simulink model "GCU_Model_genCode"  (R2018a)
settings: Solver=FixedStepDiscrete  StartTime=0.0  StopTime=20  FixedStep=0.0001  RelTol=1e-3  EnableMultiTasking=on
undefined symbols (not defined in the file): ConversionGainVector, ConversionOffsetVector, VoltageGainVector, VoltageOffsetVector
libraries: canLib x5, simulink x5, uartLib x2, utilityLib x1, clutchMotorLib x1, efiLib x1, engineControlLib x1, cstblocks x1, gearMotorLib x1
(part 1 of 3)
settings Model: Creator=SIMONE  LastModifiedBy=SIMONE
settings SolverCC: AutoInsertRateTranBlk=on
settings OptimizationCC: DefaultParameterBehavior=Inlined  UseDivisionForNetSlopeComputation=on  UseFloatMulNetSlope=on  InlineInvariantSignals=on  PassReuseOutputArgsAs=Individual arguments  ZeroExternalMemoryAtStartup=off  ZeroInternalMemoryAtStartup=off  NoFixptDivByZeroProtection=on  EfficientFloat2IntCast=on  LifeSpan=1  OptimizeBlockOrder=speed  DifferentSizesBufferReuse=on
settings DebuggingCC: ParameterTunabilityLossMsg=error
settings HardwareCC: ProdBitPerPointer=32  ProdBitPerSizeT=32  ProdBitPerPtrDiffT=32  ProdLargestAtomicInteger=Long  ProdLargestAtomicFloat=Double  ProdWordSize=32  ProdLongLongMode=on  ProdHWDeviceType=ARM Compatible->ARM Cortex
settings SFSimCC: MATLABDynamicMemAlloc=off
settings SFSimCC: SimCustomHeaderCode=|
  | #include "timings.h"
  | #include "constant_defines.h"
  | #include "id_can.h"
settings RTWCC: SystemTargetFile=ert.tlc  TemplateMakefile=ert_default_tmf  GenerateReport=on  IncludeHyperlinkInReport=on  LaunchReport=on  GenerateTraceInfo=on  GenerateTraceReport=on  GenerateTraceReportSl=on  GenerateTraceReportSf=on  GenerateTraceReportEml=on  GenerateCodeMetricsReport=on
settings RTWCC: CustomHeaderCode=|
  | #include "timings.h"
  | #include "constant_defines.h"
  | #include "id_can.h"
settings CodeAppCC: ForceParamTrailComments=on  IgnoreCustomStorageClasses=off  OperatorAnnotations=on  SimulinkDataObjDesc=on  SFDataObjDesc=on  CustomSymbolStrGlobalVar=rt$N$M  CustomSymbolStrType=$N$M  CustomSymbolStrFcn=$N$M$F  CustomSymbolStrMacro=$N$M  InsertBlockDesc=on
settings ERTTargetCC: TargetLangStandard=C99 (ISO)  GenerateSampleERTMain=on  IncludeMdlTerminateFcn=off  CombineSignalStateStructs=on  SupportComplex=off  SupportNonInlinedSFcns=on  InlinedParameterPlacement=NonHierarchical  ERTCustomFileTemplate=example_file_process.tlc  ERTFilePackagingFormat=CompactWithDataFile  MemSecPackage=Simulink

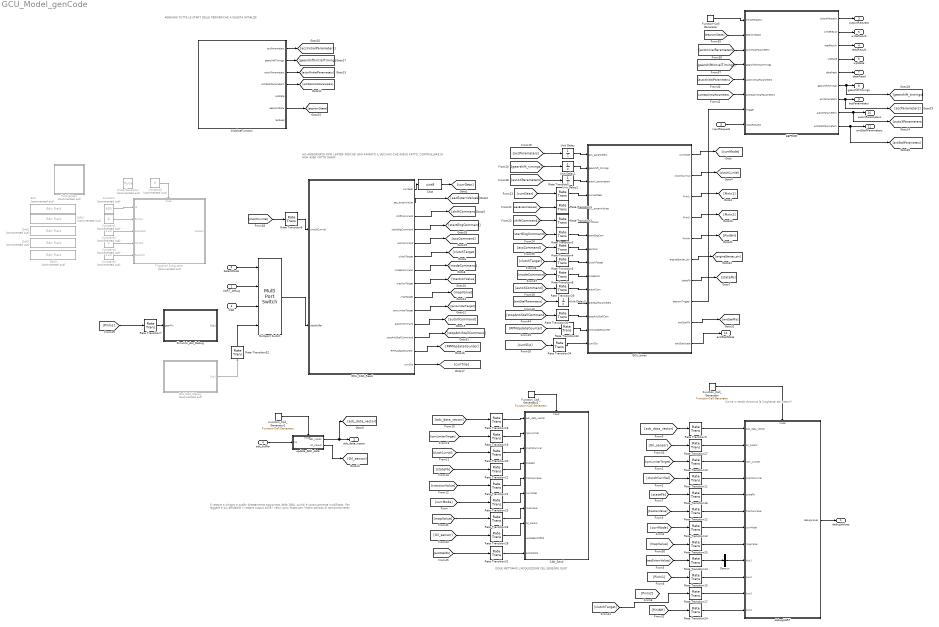
== system GCU_Model_genCode ==
  note: DOVE METTIAMO L'ACQUISIZIONE DEL SENSORE OLIO?
  note: AGGIUNGI TUTTE LE START DELLE PERIFERICHE A QUESTA INITIALIZE
  note: Il vettore a sinistra è quello direttamente aggiornato dalla DMA, quindi è continuamente modificato.
      | Per leggere è più affidabile il vettore output dove i valori sono fissati per l'intero periodo di campionamento
  note: Come si rende dinamica la lunghezza dei vettori?
  note: HO AGGIORNATO RPM_LIMITER PERCHE' ERA RIMASTO
      | IL VECCHIO CHE AVEVO FATTO, CONTROLLARE DI NON
      | AVER FATTO DANNI
  UART_debug : Inport  OutDataTypeStr=uint8  PortDimensions=10
  SelectMode : Inport  Port=2
  CAN : Inport  Port=3  OutDataTypeStr=uint8  PortDimensions=10
  adc_buffer : Inport  Port=4  OutDataTypeStr=uint32
  inputRequest : Inport  Port=5
  Anti_Stall_Debug : Subsystem  Commented=on  TreatAsAtomicUnit=on  SystemSampleTime=0.03
  CAN_Send : Subsystem  TreatAsAtomicUnit=on
  Cast : DataTypeConversion  OutDataTypeStr=uint8
  Constant : Constant  Commented=on  Value=600  OutDataTypeStr=uint16
  Constant1 : Constant  Commented=on  Value=0  OutDataTypeStr=uint16
  Constant2 : Constant  Commented=on  Value=100  OutDataTypeStr=uint16
  Constant3 : Constant  Commented=on  Value=0
  Constant4 : Constant  Commented=on  Value=0  OutDataTypeStr=uint16
  Constant5 : Constant  Commented=on  Value=100  OutDataTypeStr=uint16
  Demux : Demux  Outputs=3
  EEPROM : Subsystem
  Edit : EditField  Commented=on  WebBlockId=879  LabelPosition=Hide  Alignment=Center
  Edit1 : EditField  Commented=on  WebBlockId=880  LabelPosition=Hide  Alignment=Center
  Edit2 : EditField  Commented=on  WebBlockId=881  LabelPosition=Hide  Alignment=Center
  Edit3 : EditField  Commented=on  WebBlockId=1234  LabelPosition=Hide  Alignment=Center
  Edit4 : EditField  Commented=on  WebBlockId=1235  LabelPosition=Hide  Alignment=Center
  Function-Call Generator : simulink/Ports & Subsystems/Function-Call Generator  sample_time=[0.001,0.0009]  numberOfIterations=1
  Function_Call_Generator : simulink/Ports & Subsystems/Function-Call Generator  sample_time=[0.001, 0.0004]  numberOfIterations=1
  Function_Call_Generator1 : simulink/Ports & Subsystems/Function-Call Generator  sample_time=[0.001, 0.0006]  numberOfIterations=1
  Function_Call_Generator2 : simulink/Ports & Subsystems/Function-Call Generator  sample_time=[0.001, 0.0008]  numberOfIterations=1
  GCU_CAN_Read : Subsystem  TreatAsAtomicUnit=on  SystemSampleTime=[0.001, 0.0002]
  GCU_timer : Subsystem  TreatAsAtomicUnit=on  SystemSampleTime=0.001
  InitializeFunction : Subsystem  TreatAsAtomicUnit=on
  Multiport Switch : MultiPortSwitch  DiagnosticForDefault=Warning
  Pulse Generator : DiscretePulseGenerator  Commented=on  PulseType=Time based  Period=0.01  PulseWidth=20
  Push Button : Subsystem  Commented=on  DialogController=hmiCreateDDGDialog  IsWebBlock=on  mask(MWDashboardBlock){webBlockId=12b47424-de0c-4dac-be92-db9266863398, webBlockType=pushbutton, ShowInLibBrwoser=on, ShowInitialText=on, HMISrcModelName=GCU_Model_genCode}
      mask prompts: webBlockId "WebBlock Id"; webBlockType "WebBlock Type"; HMISrcModelName "Source Model"
      mask help: SimulinkHMI:dialogs:PushButtonDialogDesc
      mask Help: helpview([docroot '/mapfiles/simulink.map'], 'hmi_push_button')
      mask Display:
      | model = bdroot(gcb);
      | if strcmp(get_param(model,'BlockDiagramType'), 'library')
      |     image([(matlabroot) '/toolbox/simulink/hmi/icons/PushButton.png']);
      | end
  Rate Transition{,1..33} (34 alike) : RateTransition  Deterministic=off
  Rate Transition34 : RateTransition
  Simulink_Acc_Debug : Subsystem  TreatAsAtomicUnit=on  SystemSampleTime=[0.001, 0.0002]
  Triggered Subsystem : Subsystem  Commented=on  TreatAsAtomicUnit=on
  Unit Delay{,1..3} (4 alike) : UnitDelay  SampleTime=-1
  debugUART : Subsystem  TreatAsAtomicUnit=on
  update_ADC_data : Subsystem  TreatAsAtomicUnit=on
  "debugValues " : Outport
  adc_data_vector : Outport  Port=2  OutDataTypeStr=uint32
  outputRequest : Outport  Port=3
  readResult : Outport  Port=4  OutDataTypeStr=uint8  PortDimensions=1
  writeResult : Outport  Port=5  OutDataTypeStr=uint8  PortDimensions=1
  wpState : Outport  Port=6  OutDataTypeStr=uint8  PortDimensions=1
  dataRead : Outport  Port=7  OutDataTypeStr=uint8
  gearshiftTimings : Outport  Port=8
  accParameters : Outport  Port=9
  autoXParameters : Outport  Port=10
  antiStallParameters : Outport  Port=11
  antiStallState : Outport  Port=12
  wires:
  Multiport Switch/1 -> GCU_CAN_Read/2(dataBuffer)
  Rate Transition8/1 -> GCU_timer/10(modeCom)
  Rate Transition/1 -> GCU_timer/4(currentGear)
  Cast/1 -> [currGear]
  GCU_timer/3(PinIn1) -> [PinIn1]
  Rate Transition4/1 -> GCU_timer/8(aacCom)
  GCU_CAN_Read/2(aac_externValue) -> [aacExternValues]
  GCU_CAN_Read/3(shiftCommand) -> [shiftCommand]
  Rate Transition5/1 -> GCU_timer/9(clutchTarget)
  GCU_CAN_Read/1(currGear) -> Cast/1
  Rate Transition2/1 -> GCU_timer/6(shiftCom)
  Rate Transition1/1 -> GCU_timer/5(aac_externValues)
  Rate Transition3/1 -> GCU_timer/7(startEngCom)
  Function_Call_Generator/1 -> debugUART/Trigger
  debugUART/1(debugValues) -> "debugValues "/1
  Rate Transition10/1 -> debugUART/3(rpm_Limiter)
  Rate Transition11/1 -> debugUART/4(clutchCurrVal)
  GCU_timer/1(currMode) -> [currMode]
  [rpmLimiterTarget] -> Rate Transition10/1
  [clutchCurrVal] -> Rate Transition11/1
  [tractionValue] -> Rate Transition12/1
  Rate Transition12/1 -> debugUART/6(tractionValue)
  [currMode] -> Rate Transition13/1
  Rate Transition13/1 -> debugUART/7(currMode)
  [aacExternValues] -> Rate Transition14/1
  Constant/1 -> Triggered Subsystem/1(id)
  Constant2/1 -> Triggered Subsystem/3(secondInt)
  Constant1/1 -> Triggered Subsystem/2(firstInt)
  SelectMode/1 -> Multiport Switch/1
  GCU_timer/7(stateFb) -> [stateFb]
  [stateFb] -> Rate Transition16/1
  Rate Transition16/1 -> debugUART/5(stateFb)
  Function_Call_Generator1/1 -> update_ADC_data/Trigger
  adc_buffer/1 -> update_ADC_data/1(In1)
  update_ADC_data/1(adc_inputs) -> [adc_data_vector], adc_data_vector/1
  [adc_data_vector] -> Rate Transition9/1
  Rate Transition9/1 -> debugUART/1(adc_data_vector)
  Function_Call_Generator2/1 -> CAN_Send/Trigger
  [adc_data_vector] -> Rate Transition18/1
  GCU_CAN_Read/8(tractionTarget) -> [tractionValue]
  [currMode] -> Rate Transition23/1
  [clutchCurrVal] -> Rate Transition20/1
  [tractionValue] -> Rate Transition22/1
  [rpmLimiterTarget] -> Rate Transition19/1
  [stateFb] -> Rate Transition21/1
  Rate Transition18/1 -> CAN_Send/1(adc_data_vector)
  Rate Transition19/1 -> CAN_Send/2(rpmLimiter)
  Rate Transition20/1 -> CAN_Send/3(clutchCurrVal)
  Rate Transition21/1 -> CAN_Send/4(stateFb)
  Rate Transition22/1 -> CAN_Send/5(tractionValue)
  Rate Transition23/1 -> CAN_Send/6(currMode)
  InitializeFunction/1(accParameters) -> [accInitialParameters]
  InitializeFunction/2(gearshiftTimings) -> [gearshiftInitialTimings]
  Constant3/1 -> Triggered Subsystem/Trigger
  Constant4/1 -> Triggered Subsystem/4(thirdInt)
  Constant5/1 -> Triggered Subsystem/5(fourthInt)
  [aacExternValues] -> Rate Transition1/1
  [shiftCommand] -> Rate Transition2/1
  [currGear] -> Rate Transition/1
  GCU_CAN_Read/4(startEngCommand) -> [startEngCommand]
  [startEngCommand] -> Rate Transition3/1
  GCU_CAN_Read/5(accCommand) -> [accCommand]
  [accCommand] -> Rate Transition4/1
  GCU_CAN_Read/6(clutchTarget) -> [clutchTarget]
  [clutchTarget] -> Rate Transition5/1
  GCU_CAN_Read/7(modeCommand) -> [modeCommand]
  [modeCommand] -> Rate Transition8/1
  [clutchCurrVal] -> Rate Transition6/1
  Rate Transition6/1 -> GCU_CAN_Read/1(clutchCurrVal)
  [PinIn1] -> Rate Transition7/1
  Rate Transition7/1 -> Simulink_Acc_Debug/1(gearPin)
  Rate Transition14/1 -> Demux/1
  Demux/2 -> debugUART/9(Aux1)
  Rate Transition15/1 -> debugUART/10(Aux2)
  [PinIn1] -> Rate Transition15/1
  Rate Transition17/1 -> debugUART/11(Aux3)
  GCU_timer/4(PinIn2) -> [PinIn2]
  GCU_timer/5(PinINH) -> [PinINH]
  [PinINH] -> Rate Transition24/1
  Rate Transition24/1 -> debugUART/12(Aux4)
  GCU_timer/6(engineStarter_pin) -> [engineStarter_pin]
  [mapValue] -> Rate Transition25/1
  Rate Transition25/1 -> debugUART/8(mapValue)
  GCU_CAN_Read/9(mapTarget) -> [mapValue]
  [mapValue] -> Rate Transition26/1
  Rate Transition26/1 -> CAN_Send/7(mapValue)
  update_ADC_data/2(oil_sensor) -> [Oil_sensor]
  [Oil_sensor] -> Rate Transition27/1
  Rate Transition27/1 -> debugUART/2(oil_sensor)
  [Oil_sensor] -> Rate Transition28/1
  Rate Transition28/1 -> CAN_Send/8(oil_sensor)
  CAN/1 -> Multiport Switch/3
  UART_debug/1 -> Multiport Switch/2
  EEPROM/1(outputRequest) -> outputRequest/1
  inputRequest/1 -> EEPROM/8(inputRequest)
  EEPROM/2(writeResult) -> writeResult/1
  EEPROM/3(readResult) -> readResult/1
  EEPROM/4(wpState) -> wpState/1
  EEPROM/5(dataRead) -> dataRead/1
  InitializeFunction/6(eepromState) -> [eepromState]
  [eepromState] -> EEPROM/2(eepromState)
  [accInitialParameters] -> EEPROM/3(accInitialParameters)
  [gearshiftInitialTimings] -> EEPROM/4(gearshiftInitialTimings)
  EEPROM/6(gearshiftTimings) -> [gearshift_timings], gearshiftTimings/1
  EEPROM/7(accParameters) -> [accParameters], accParameters/1
  GCU_CAN_Read/10(rpmLimiterTarget) -> [rpmLimiterTarget]
  [accParameters] -> Unit Delay/1
  [gearshift_timings] -> Unit Delay1/1
  InitializeFunction/3(autoXParameters) -> [autoXInitialParameters]
  EEPROM/8(autoXParameters) -> [autoXParameters], autoXParameters/1
  [autoXParameters] -> Unit Delay2/1
  GCU_CAN_Read/11(autoXCommand) -> [autoXCommand]
  [autoXCommand] -> Rate Transition29/1
  Rate Transition29/1 -> GCU_timer/11(autoXCom)
  Function-Call Generator/1 -> EEPROM/1(serialRequest)
  [autoXInitialParameters] -> EEPROM/5(autoXInitialParameters)
  GCU_timer/2(clutchCurrVal) -> [clutchCurrVal]
  [clutchTarget] -> Rate Transition17/1
  InitializeFunction/4(antiStallParameters) -> [antiStallInitialParameters]
  [antiStallInitialParameters] -> EEPROM/6(antiStallInitialParameters)
  EEPROM/9(antiStallParameters) -> [antiStallParameters], antiStallParameters/1
  [antiStallParameters] -> Unit Delay3/1
  GCU_CAN_Read/12(stopAntiStallCommand) -> [stopAntiStallCommand]
  [stopAntiStallCommand] -> Rate Transition30/1
  Rate Transition30/1 -> GCU_timer/13(stopAntiStallCom)
  GCU_timer/8(eepromTrigger) -> EEPROM/7(Trigger)
  Unit Delay/1 -> GCU_timer/1(acc_parameters)
  Unit Delay1/1 -> GCU_timer/2(gearshift_timings)
  Unit Delay2/1 -> GCU_timer/3(autoX_parameters)
  GCU_timer/9(antiStallFb) -> [antiStallFb]
  [antiStallFb] -> Rate Transition31/1
  Rate Transition31/1 -> CAN_Send/10(antiStallFb)
  Unit Delay3/1 -> GCU_timer/12(antiStallParameters)
  Anti_Stall_Debug/1(Out1) -> Rate Transition32/1
  GCU_CAN_Read/13(RPMUpdateCounter) -> [RPMUpdateCounter]
  [RPMUpdateCounter] -> Rate Transition33/1
  Rate Transition33/1 -> GCU_timer/14(rpmUpdateCounter)
  GCU_timer/10(antiStallstate) -> antiStallState/1
  Rate Transition32/1 -> Multiport Switch/4
  GCU_CAN_Read/14(currSlip) -> [currSlip]
  [currSlip] -> Rate Transition34/1
  Rate Transition34/1 -> GCU_timer/15(currSlip)

== system GCU_Model_genCode/Anti_Stall_Debug ==
  AccelerationRoutine : Stateflow chart  TreatAsAtomicUnit=on
  PackCanUart : S-Function  FunctionName=PackCanUART  SFunctionDeploymentMode=off  EnableBusSupport=off
  Out1 : Outport
  wires:
  PackCanUart/1 -> Out1/1
  AccelerationRoutine/2(firstInt) -> PackCanUart/2
  AccelerationRoutine/1(id) -> PackCanUart/1
  AccelerationRoutine/3(secondInt) -> PackCanUart/3
  AccelerationRoutine/4(thirdInt) -> PackCanUart/4

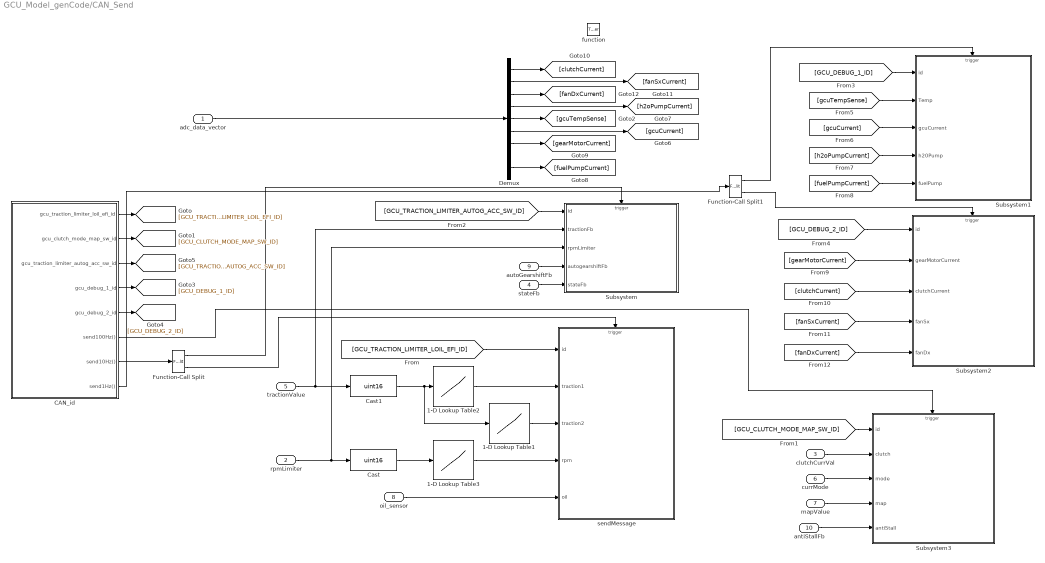
== system GCU_Model_genCode/CAN_Send ==
  adc_data_vector : Inport
  rpmLimiter : Inport  Port=2
  clutchCurrVal : Inport  Port=3
  stateFb : Inport  Port=4
  tractionValue : Inport  Port=5
  currMode : Inport  Port=6
  mapValue : Inport  Port=7
  oil_sensor : Inport  Port=8
  autoGearshiftFb : Inport  Port=9
  antiStallFb : Inport  Port=10
  function : TriggerPort  TriggerType=function-call  VariantControl=Variant
  1-D Lookup Table1 : Lookup_n-D  NumberOfTableDimensions=1  BreakpointsForDimension1=[0:7]  Table=[uint16(0),uint16(100),uint16(200),uint16(300),uint16(400),uint16(500),uint16(600),uint16(700)]  ExtrapMethod=Clip  InternalRulePriority=Speed  RndMeth=Simplest  InputSameDT=on
  1-D Lookup Table2 : Lookup_n-D  NumberOfTableDimensions=1  BreakpointsForDimension1=[0:7]  Table=[uint16(0),uint16(100),uint16(200),uint16(300),uint16(400),uint16(500),uint16(600),uint16(700)]  ExtrapMethod=Clip  InternalRulePriority=Speed  RndMeth=Simplest  InputSameDT=on
  1-D Lookup Table3 : Lookup_n-D  NumberOfTableDimensions=1  BreakpointsForDimension1=[65,70,75,80,85,90,95,100,105,110,115]  Table=[uint16(0),uint16(100),uint16(200),uint16(300),uint16(400),uint16(500),uint16(600),uint16(700),uint16(800),uint16(900),uint16(1000)];  ExtrapMethod=Clip  InternalRulePriority=Speed  RndMeth=Simplest  InputSameDT=on
  CAN_id : Stateflow chart  TreatAsAtomicUnit=on
  Cast : DataTypeConversion  OutDataTypeStr=uint16
  Cast1 : DataTypeConversion  OutDataTypeStr=uint16
  Demux : Demux  Outputs=9
  Function-Call Split : FunctionCallSplit  IconShape=distinctive  NumOutputPorts=2  OutputPortLayout=default
  Function-Call Split1 : FunctionCallSplit  IconShape=distinctive  NumOutputPorts=2  OutputPortLayout=default
  Subsystem : Subsystem
  Subsystem1 : Subsystem
  Subsystem2 : Subsystem
  Subsystem3 : Subsystem
  sendMessage : Subsystem
  wires:
  adc_data_vector/1 -> Demux/1
  CAN_id/1(gcu_traction_limiter_loil_efi_id) -> [GCU_TRACTION_LIMITER_LOIL_EFI_ID]
  CAN_id/2(gcu_clutch_mode_map_sw_id) -> [GCU_CLUTCH_MODE_MAP_SW_ID]
  CAN_id/3(gcu_traction_limiter_autog_acc_sw_id) -> [GCU_TRACTION_LIMITER_AUTOG_ACC_SW_ID]
  CAN_id/4(gcu_debug_1_id) -> [GCU_DEBUG_1_ID]
  CAN_id/5(gcu_debug_2_id) -> [GCU_DEBUG_2_ID]
  tractionValue/1 -> Subsystem/2(tractionFb), Cast1/1
  rpmLimiter/1 -> Subsystem/3(rpmLimiter), Cast/1
  Demux/5 -> [gcuTempSense]
  Demux/6 -> [gcuCurrent]
  Demux/4 -> [h2oPumpCurrent]
  Demux/9 -> [fuelPumpCurrent]
  Demux/7 -> [gearMotorCurrent]
  Demux/1 -> [clutchCurrent]
  Demux/2 -> [fanSxCurrent]
  Demux/3 -> [fanDxCurrent]
  Cast/1 -> 1-D Lookup Table3/1
  Cast1/1 -> 1-D Lookup Table1/1, 1-D Lookup Table2/1
  [GCU_TRACTION_LIMITER_LOIL_EFI_ID] -> sendMessage/1(id)
  1-D Lookup Table2/1 -> sendMessage/2(traction1)
  1-D Lookup Table1/1 -> sendMessage/3(traction2)
  1-D Lookup Table3/1 -> sendMessage/4(rpm)
  oil_sensor/1 -> sendMessage/5(oil)
  [GCU_TRACTION_LIMITER_AUTOG_ACC_SW_ID] -> Subsystem/1(id)
  autoGearshiftFb/1 -> Subsystem/4(autogearshiftFb)
  stateFb/1 -> Subsystem/5(stateFb)
  [GCU_DEBUG_1_ID] -> Subsystem1/1(id)
  [gcuTempSense] -> Subsystem1/2(Temp)
  [gcuCurrent] -> Subsystem1/3(gcuCurrent)
  [h2oPumpCurrent] -> Subsystem1/4(h20Pump)
  [fuelPumpCurrent] -> Subsystem1/5(fuelPump)
  [GCU_DEBUG_2_ID] -> Subsystem2/1(id)
  [gearMotorCurrent] -> Subsystem2/2(gearMotorCurrent)
  [clutchCurrent] -> Subsystem2/3(clutchCurrent)
  [fanSxCurrent] -> Subsystem2/4(fanSx)
  [fanDxCurrent] -> Subsystem2/5(fanDx)
  [GCU_CLUTCH_MODE_MAP_SW_ID] -> Subsystem3/1(id)
  clutchCurrVal/1 -> Subsystem3/2(clutch)
  currMode/1 -> Subsystem3/3(mode)
  mapValue/1 -> Subsystem3/4(map)
  antiStallFb/1 -> Subsystem3/5(antiStall)
  CAN_id/6(send100Hz()) -> Subsystem3/Trigger
  CAN_id/7(send10Hz()) -> Function-Call Split/1
  Function-Call Split/1 -> Subsystem/Trigger
  Function-Call Split/2 -> sendMessage/Trigger
  CAN_id/8(send1Hz()) -> Function-Call Split1/1
  Function-Call Split1/2 -> Subsystem2/Trigger
  Function-Call Split1/1 -> Subsystem1/Trigger

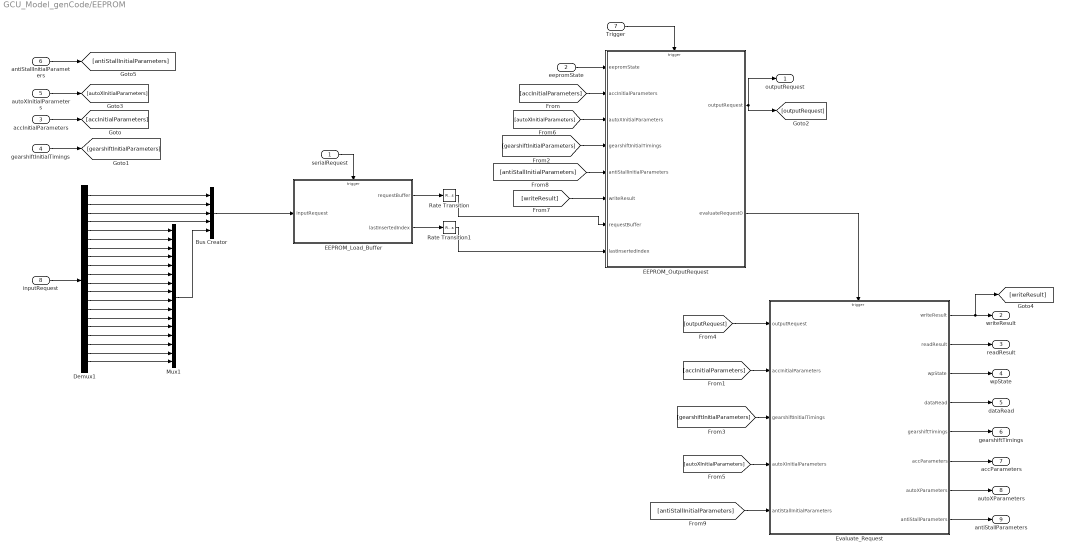
== system GCU_Model_genCode/EEPROM ==
  serialRequest : Inport
  eepromState : Inport  Port=2
  accInitialParameters : Inport  Port=3
  gearshiftInitialTimings : Inport  Port=4
  autoXInitialParameters : Inport  Port=5
  antiStallInitialParameters : Inport  Port=6
  Trigger : Inport  Port=7
  inputRequest : Inport  Port=8  OutDataTypeStr=uint8  PortDimensions=[1,20]
  Bus Creator : BusCreator  Inputs=5  OutDataTypeStr=Bus: eepromRequest
      settings: InheritFromInputs=off
  Demux1 : Demux  Outputs=20
  EEPROM_Load_Buffer : Stateflow chart  TreatAsAtomicUnit=on
  EEPROM_OutputRequest : Stateflow chart  TreatAsAtomicUnit=on
  Evaluate_Request : Subsystem  TreatAsAtomicUnit=on
  Mux1 : Mux  Inputs=16
  Rate Transition : RateTransition  Deterministic=off  OutPortSampleTime=0.001
  Rate Transition1 : RateTransition  Deterministic=off  InitialCondition=1  OutPortSampleTime=0.001
  outputRequest : Outport
  writeResult : Outport  Port=2
  readResult : Outport  Port=3
  wpState : Outport  Port=4  OutDataTypeStr=uint8
  dataRead : Outport  Port=5
  gearshiftTimings : Outport  Port=6
  accParameters : Outport  Port=7
  autoXParameters : Outport  Port=8
  antiStallParameters : Outport  Port=9
  wires:
  Mux1/1 -> Bus Creator/5
  Demux1/19 -> Mux1/15
  Demux1/20 -> Mux1/16
  Demux1/2 -> Bus Creator/2
  inputRequest/1 -> Demux1/1
  Demux1/13 -> Mux1/9
  Demux1/16 -> Mux1/12
  Demux1/11 -> Mux1/7
  Demux1/15 -> Mux1/11
  Demux1/7 -> Mux1/3
  Demux1/14 -> Mux1/10
  Demux1/10 -> Mux1/6
  Demux1/17 -> Mux1/13
  Demux1/3 -> Bus Creator/3
  Demux1/4 -> Bus Creator/4
  Demux1/8 -> Mux1/4
  Demux1/12 -> Mux1/8
  Demux1/1 -> Bus Creator/1
  Bus Creator/1 -> EEPROM_Load_Buffer/1(inputRequest)
  serialRequest/1 -> EEPROM_Load_Buffer/Trigger
  Demux1/6 -> Mux1/2
  Demux1/18 -> Mux1/14
  Demux1/9 -> Mux1/5
  Demux1/5 -> Mux1/1
  Trigger/1 -> EEPROM_OutputRequest/Trigger
  Rate Transition/1 -> EEPROM_OutputRequest/7(requestBuffer)
  Rate Transition1/1 -> EEPROM_OutputRequest/8(lastInsertedIndex)
  EEPROM_OutputRequest/2(evaluateRequest()) -> Evaluate_Request/Trigger
  Evaluate_Request/1(writeResult) -> [writeResult], writeResult/1
  Evaluate_Request/2(readResult) -> readResult/1
  Evaluate_Request/3(wpState) -> wpState/1
  Evaluate_Request/4(dataRead) -> dataRead/1
  EEPROM_Load_Buffer/1(requestBuffer) -> Rate Transition/1
  EEPROM_Load_Buffer/2(lastInsertedIndex) -> Rate Transition1/1
  eepromState/1 -> EEPROM_OutputRequest/1(eepromState)
  Evaluate_Request/5(gearshiftTimings) -> gearshiftTimings/1
  Evaluate_Request/6(accParameters) -> accParameters/1
  accInitialParameters/1 -> [accInitialParameters]
  [accInitialParameters] -> EEPROM_OutputRequest/2(accInitialParameters)
  [accInitialParameters] -> Evaluate_Request/2(accInitialParameters)
  gearshiftInitialTimings/1 -> [gearshiftInitialParameters]
  [gearshiftInitialParameters] -> EEPROM_OutputRequest/4(gearshiftInitialTimings)
  [gearshiftInitialParameters] -> Evaluate_Request/3(gearshiftInitialTimings)
  EEPROM_OutputRequest/1(outputRequest) -> [outputRequest], outputRequest/1
  [outputRequest] -> Evaluate_Request/1(outputRequest)
  Evaluate_Request/7(autoXParameters) -> autoXParameters/1
  autoXInitialParameters/1 -> [autoXInitialParameters]
  [autoXInitialParameters] -> Evaluate_Request/4(autoXInitialParameters)
  [autoXInitialParameters] -> EEPROM_OutputRequest/3(autoXInitialParameters)
  [writeResult] -> EEPROM_OutputRequest/6(writeResult)
  antiStallInitialParameters/1 -> [antiStallInitialParameters]
  [antiStallInitialParameters] -> EEPROM_OutputRequest/5(antiStallInitialParameters)
  [antiStallInitialParameters] -> Evaluate_Request/5(antiStallInitialParameters)
  Evaluate_Request/8(antiStallParameters) -> antiStallParameters/1

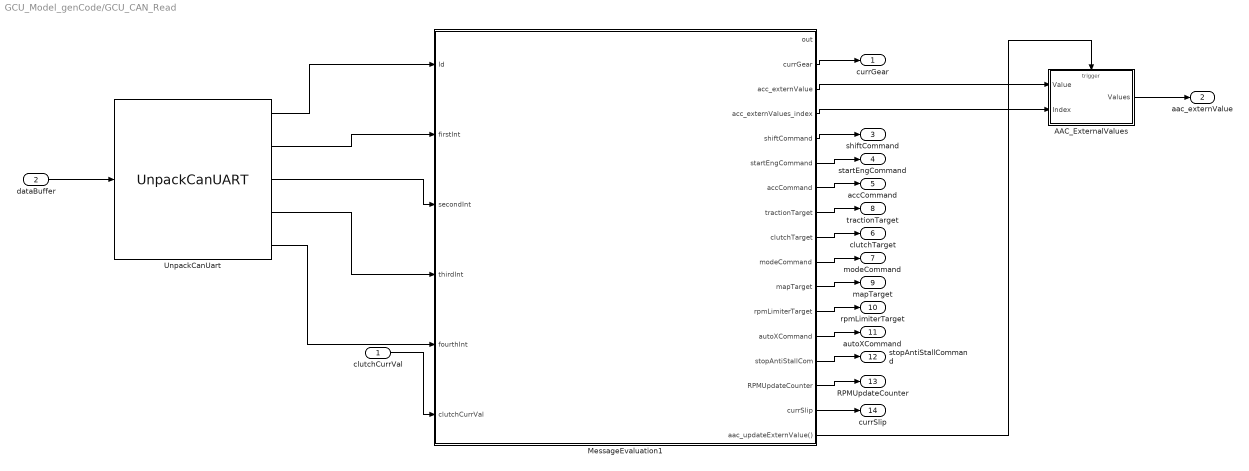
== system GCU_Model_genCode/GCU_CAN_Read ==
  clutchCurrVal : Inport
  dataBuffer : Inport  Port=2
  AAC_ExternalValues : Subsystem  TreatAsAtomicUnit=on
  MessageEvaluation1 : Stateflow chart  TreatAsAtomicUnit=on
  UnpackCanUart : S-Function  FunctionName=UnpackCanUART  SFunctionDeploymentMode=off  EnableBusSupport=off
  currGear : Outport
  aac_externValue : Outport  Port=2
  shiftCommand : Outport  Port=3
  startEngCommand : Outport  Port=4
  accCommand : Outport  Port=5
  clutchTarget : Outport  Port=6
  modeCommand : Outport  Port=7
  tractionTarget : Outport  Port=8
  mapTarget : Outport  Port=9
  rpmLimiterTarget : Outport  Port=10
  autoXCommand : Outport  Port=11
  stopAntiStallCommand : Outport  Port=12
  RPMUpdateCounter : Outport  Port=13
  currSlip : Outport  Port=14
  wires:
  UnpackCanUart/4 -> MessageEvaluation1/4(thirdInt)
  MessageEvaluation1/4(acc_externValues_index) -> AAC_ExternalValues/2(Index)
  MessageEvaluation1/7(accCommand) -> accCommand/1
  MessageEvaluation1/9(clutchTarget) -> clutchTarget/1
  dataBuffer/1 -> UnpackCanUart/1
  MessageEvaluation1/10(modeCommand) -> modeCommand/1
  MessageEvaluation1/5(shiftCommand) -> shiftCommand/1
  MessageEvaluation1/3(acc_externValue) -> AAC_ExternalValues/1(Value)
  MessageEvaluation1/6(startEngCommand) -> startEngCommand/1
  UnpackCanUart/1 -> MessageEvaluation1/1(Id)
  UnpackCanUart/5 -> MessageEvaluation1/5(fourthInt)
  UnpackCanUart/3 -> MessageEvaluation1/3(secondInt)
  clutchCurrVal/1 -> MessageEvaluation1/6(clutchCurrVal)
  MessageEvaluation1/2(currGear) -> currGear/1
  MessageEvaluation1/17(aac_updateExternValue()) -> AAC_ExternalValues/Trigger
  UnpackCanUart/2 -> MessageEvaluation1/2(firstInt)
  AAC_ExternalValues/1(Values) -> aac_externValue/1
  MessageEvaluation1/11(mapTarget) -> mapTarget/1
  MessageEvaluation1/8(tractionTarget) -> tractionTarget/1
  MessageEvaluation1/12(rpmLimiterTarget) -> rpmLimiterTarget/1
  MessageEvaluation1/13(autoXCommand) -> autoXCommand/1
  MessageEvaluation1/14(stopAntiStallCom) -> stopAntiStallCommand/1
  MessageEvaluation1/15(RPMUpdateCounter) -> RPMUpdateCounter/1
  MessageEvaluation1/16(currSlip) -> currSlip/1

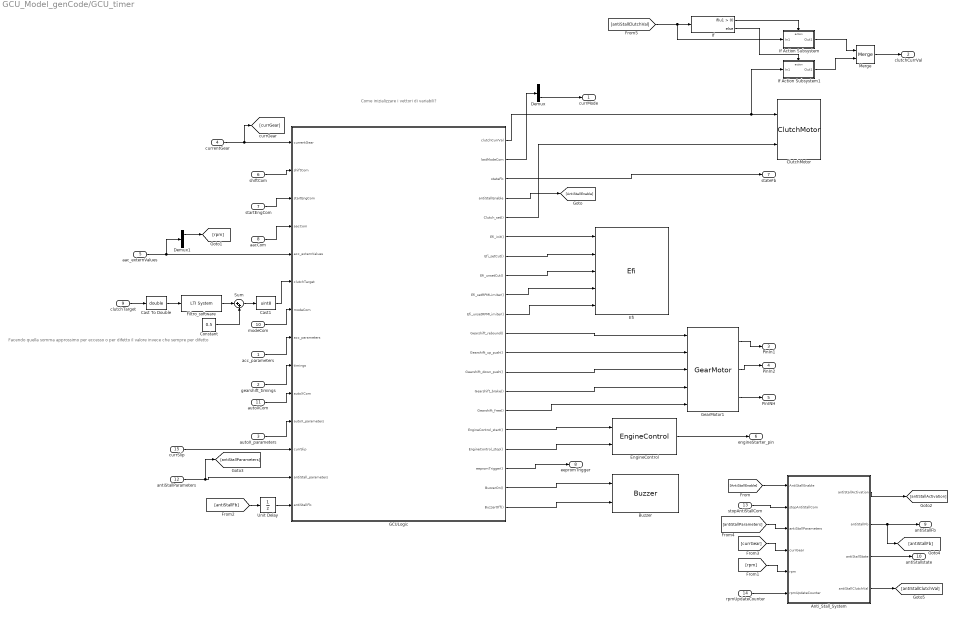
== system GCU_Model_genCode/GCU_timer ==
  note: Facendo quella somma approssimo per eccesso o per difetto il valore
      | invece che sempre per difetto
  note: Come inizializzare i vettori di variabili?
  acc_parameters : Inport
  gearshift_timings : Inport  Port=2
  autoX_parameters : Inport  Port=3
  currentGear : Inport  Port=4
  aac_externValues : Inport  Port=5
  shiftCom : Inport  Port=6
  startEngCom : Inport  Port=7
  aacCom : Inport  Port=8
  clutchTarget : Inport  Port=9
  modeCom : Inport  Port=10
  autoXCom : Inport  Port=11
  antiStallParameters : Inport  Port=12
  stopAntiStallCom : Inport  Port=13
  rpmUpdateCounter : Inport  Port=14
  currSlip : Inport  Port=15
  Anti_Stall_System : Subsystem  TreatAsAtomicUnit=on
  Buzzer : utilityLib/Buzzer
      settings: SourceProductName=GCU Library
  Cast To Double : DataTypeConversion  OutDataTypeStr=double
  Cast1 : DataTypeConversion  OutDataTypeStr=uint8
  ClutchMotor : clutchMotorLib/ClutchMotor
      settings: SourceProductName=GCU Library
  Constant : Constant  Value=0.5  OutDataTypeStr=uint8
  Demux : Demux  Outputs=2
  Demux1 : Demux  Outputs=3
  Efi : efiLib/Efi
      settings: SourceProductName=GCU Library
  EngineControl : engineControlLib/EngineControl
      settings: SourceProductName=GCU Library
  Filtro_software : cstblocks/LTI System  sys=F_z  IC=[]
  GCULogic : Stateflow chart  TreatAsAtomicUnit=on
  GearMotor1 : gearMotorLib/GearMotor
      settings: SourceProductName=GCU Library
  If : If
  If Action Subsystem : Subsystem  TreatAsAtomicUnit=on
  If Action Subsystem1 : Subsystem  TreatAsAtomicUnit=on
  Merge : Merge
  Sum : Sum  Inputs=|++
  Unit Delay : UnitDelay  SampleTime=-1
  currMode : Outport
  clutchCurrVal : Outport  Port=2
  PinIn1 : Outport  Port=3
  PinIn2 : Outport  Port=4
  PinINH : Outport  Port=5
  engineStarter_pin : Outport  Port=6
  stateFb : Outport  Port=7
  eepromTrigger : Outport  Port=8
  antiStallFb : Outport  Port=9
  antiStallstate : Outport  Port=10
  wires:
  GCULogic/17(EngineControl_stop()) -> EngineControl/2
  startEngCom/1 -> GCULogic/3(startEngCom)
  GCULogic/9(Efi_setRPMLimiter()) -> Efi/4
  GCULogic/6(Efi_init()) -> Efi/1
  GCULogic/16(EngineControl_start()) -> EngineControl/1
  GearMotor1/3 -> PinINH/1
  GCULogic/10(Efi_unsetRPMLimiter()) -> Efi/5
  EngineControl/1 -> engineStarter_pin/1
  GCULogic/15(Gearshift_free()) -> GearMotor1/5
  GCULogic/14(Gearshift_brake()) -> GearMotor1/4
  GCULogic/11(Gearshift_rebound()) -> GearMotor1/1
  GearMotor1/2 -> PinIn2/1
  GearMotor1/1 -> PinIn1/1
  GCULogic/12(Gearshift_up_push()) -> GearMotor1/2
  shiftCom/1 -> GCULogic/2(shiftCom)
  aacCom/1 -> GCULogic/4(aacCom)
  GCULogic/7(Efi_setCut()) -> Efi/2
  currentGear/1 -> [currGear], GCULogic/1(currentGear)
  GCULogic/8(Efi_unsetCut()) -> Efi/3
  modeCom/1 -> GCULogic/7(modeCom)
  aac_externValues/1 -> GCULogic/5(acc_externValues), Demux1/1
  GCULogic/13(Gearshift_down_push()) -> GearMotor1/3
  GCULogic/3(stateFb) -> stateFb/1
  GCULogic/2(lastModeCom) -> Demux/1
  Demux/2 -> currMode/1
  acc_parameters/1 -> GCULogic/8(acc_parameters)
  gearshift_timings/1 -> GCULogic/9(timings)
  GCULogic/5(Clutch_set()) -> ClutchMotor/2
  GCULogic/18(eepromTrigger()) -> eepromTrigger/1
  autoXCom/1 -> GCULogic/10(autoXCom)
  autoX_parameters/1 -> GCULogic/11(autoX_parameters)
  GCULogic/19(BuzzerOn()) -> Buzzer/1
  GCULogic/20(BuzzerOff()) -> Buzzer/2
  Cast To Double/1 -> Filtro_software/1
  Cast1/1 -> GCULogic/6(clutchTarget)
  clutchTarget/1 -> Cast To Double/1
  Sum/1 -> Cast1/1
  Filtro_software/1 -> Sum/1
  Constant/1 -> Sum/2
  GCULogic/4(antiStallEnable) -> [AntiStallEnable]
  [AntiStallEnable] -> Anti_Stall_System/1(AntiStallEnable)
  stopAntiStallCom/1 -> Anti_Stall_System/2(stopAntiStallCom)
  [antiStallParameters] -> Anti_Stall_System/3(antiStallParameters)
  Demux1/1 -> [rpm]
  [rpm] -> Anti_Stall_System/5(rpm)
  Anti_Stall_System/1(antiStallActivation) -> [antiStallActivation]
  Anti_Stall_System/2(antiStallFb) -> [antiStallFb], antiStallFb/1
  [currGear] -> Anti_Stall_System/4(currGear)
  antiStallParameters/1 -> [antiStallParameters], GCULogic/13(antiStall_parameters)
  rpmUpdateCounter/1 -> Anti_Stall_System/6(rpmUpdateCounter)
  Anti_Stall_System/3(antiStallState) -> antiStallstate/1
  [antiStallFb] -> Unit Delay/1
  Unit Delay/1 -> GCULogic/14(antiStallFb)
  Anti_Stall_System/4(antiStallClutchVal) -> [antiStallClutchVal]
  GCULogic/1(clutchCurrVal) -> If Action Subsystem1/1(In1), ClutchMotor/1
  [antiStallClutchVal] -> If Action Subsystem/1(In1), If/1
  If/1 -> If Action Subsystem/Action
  If Action Subsystem1/1(Out1) -> Merge/2
  If Action Subsystem/1(Out1) -> Merge/1
  Merge/1 -> clutchCurrVal/1
  If/2 -> If Action Subsystem1/Action
  currSlip/1 -> GCULogic/12(currSlip)

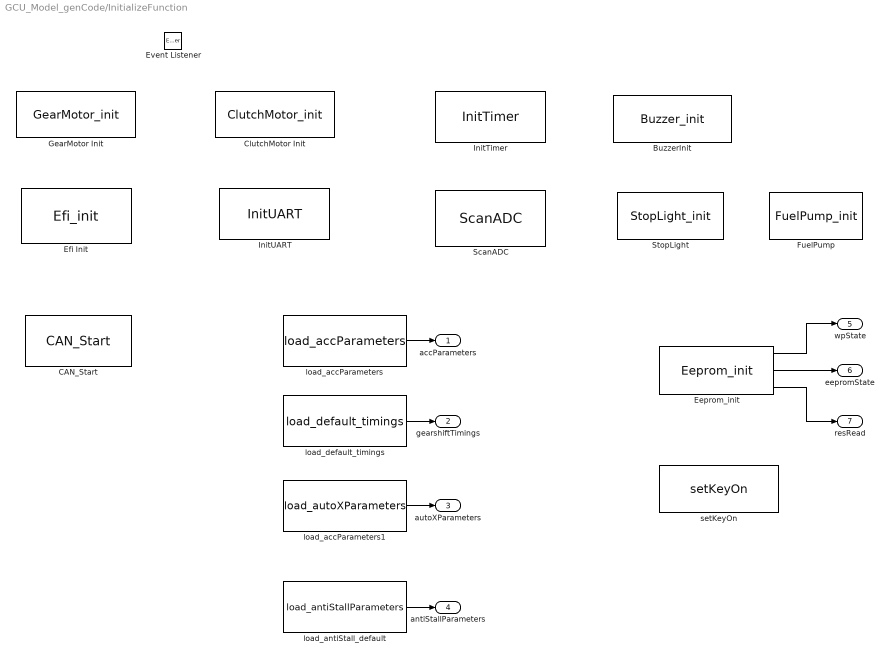
== system GCU_Model_genCode/InitializeFunction ==
  BuzzerInit : S-Function  FunctionName=Buzzer_init  SFunctionDeploymentMode=off  EnableBusSupport=off
  CAN_Start : S-Function  FunctionName=CAN_Start  SFunctionDeploymentMode=off  EnableBusSupport=off
  ClutchMotor Init : S-Function  FunctionName=ClutchMotor_init  SFunctionDeploymentMode=off  EnableBusSupport=off
  Eeprom_init : S-Function  FunctionName=Eeprom_init  SFunctionDeploymentMode=off  EnableBusSupport=off
  Efi Init : S-Function  FunctionName=Efi_init  SFunctionDeploymentMode=off  EnableBusSupport=off
  Event Listener : EventListener  DisableCoverage=on  EventName=reset
  FuelPump : S-Function  FunctionName=FuelPump_init  SFunctionDeploymentMode=off  EnableBusSupport=off
  GearMotor Init : S-Function  FunctionName=GearMotor_init  SFunctionDeploymentMode=off  EnableBusSupport=off
  InitTimer : S-Function  FunctionName=InitTimer  SFunctionDeploymentMode=off  EnableBusSupport=off
  InitUART : S-Function  FunctionName=InitUART  SFunctionDeploymentMode=off  EnableBusSupport=off
  ScanADC : S-Function  FunctionName=ScanADC  SFunctionDeploymentMode=off  EnableBusSupport=off
  StopLight : S-Function  FunctionName=StopLight_init  SFunctionDeploymentMode=off  EnableBusSupport=off
  load_accParameters : S-Function  FunctionName=load_accParameters  SFunctionDeploymentMode=off  EnableBusSupport=off
  load_accParameters1 : S-Function  FunctionName=load_autoXParameters  SFunctionDeploymentMode=off  EnableBusSupport=off
  load_antiStall_default : S-Function  FunctionName=load_antiStallParameters  SFunctionDeploymentMode=off  EnableBusSupport=off
  load_default_timings : S-Function  FunctionName=load_default_timings  SFunctionDeploymentMode=off  EnableBusSupport=off
  setKeyOn : S-Function  FunctionName=setKeyOn  SFunctionDeploymentMode=off  EnableBusSupport=off
  accParameters : Outport
  gearshiftTimings : Outport  Port=2
  autoXParameters : Outport  Port=3
  antiStallParameters : Outport  Port=4
  wpState : Outport  Port=5
  eepromState : Outport  Port=6
  resRead : Outport  Port=7
  wires:
  load_accParameters/1 -> accParameters/1
  load_default_timings/1 -> gearshiftTimings/1
  Eeprom_init/1 -> wpState/1
  Eeprom_init/2 -> eepromState/1
  Eeprom_init/3 -> resRead/1
  load_accParameters1/1 -> autoXParameters/1
  load_antiStall_default/1 -> antiStallParameters/1

== system GCU_Model_genCode/Push Button ==

== system GCU_Model_genCode/Simulink_Acc_Debug ==
  gearPin : Inport
  AccelerationRoutine : Stateflow chart  TreatAsAtomicUnit=on  SystemSampleTime=[0.001, 0.0002]
  PackCanUart : S-Function  FunctionName=PackCanUART  SFunctionDeploymentMode=off  EnableBusSupport=off
  Out1 : Outport
  wires:
  PackCanUart/1 -> Out1/1
  AccelerationRoutine/2(firstInt) -> PackCanUart/2
  AccelerationRoutine/1(id) -> PackCanUart/1
  AccelerationRoutine/3(secondInt) -> PackCanUart/3
  gearPin/1 -> AccelerationRoutine/1(gearPin)
  AccelerationRoutine/4(thirdInt) -> PackCanUart/4

== system GCU_Model_genCode/Triggered Subsystem ==
  id : Inport
  firstInt : Inport  Port=2
  secondInt : Inport  Port=3
  thirdInt : Inport  Port=4
  fourthInt : Inport  Port=5
  Trigger : TriggerPort  VariantControl=Variant
  PackCanUart : S-Function  FunctionName=PackCanUART  SFunctionDeploymentMode=off  EnableBusSupport=off
  Scope : Scope
  Outport : Outport
  wires:
  PackCanUart/1 -> Outport/1, Scope/1
  id/1 -> PackCanUart/1
  firstInt/1 -> PackCanUart/2
  secondInt/1 -> PackCanUart/3
  fourthInt/1 -> PackCanUart/5
  thirdInt/1 -> PackCanUart/4

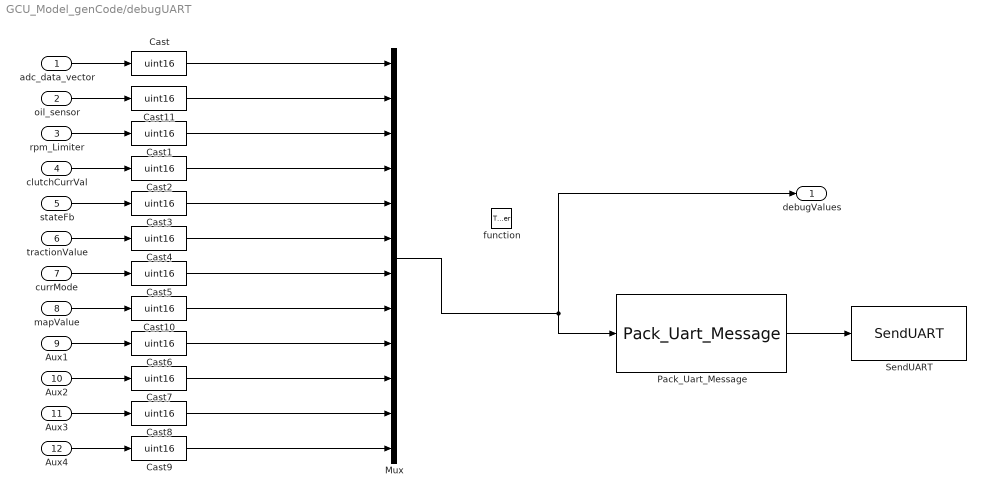
== system GCU_Model_genCode/debugUART ==
  adc_data_vector : Inport
  oil_sensor : Inport  Port=2
  rpm_Limiter : Inport  Port=3
  clutchCurrVal : Inport  Port=4
  stateFb : Inport  Port=5
  tractionValue : Inport  Port=6
  currMode : Inport  Port=7
  mapValue : Inport  Port=8
  Aux1 : Inport  Port=9
  Aux2 : Inport  Port=10
  Aux3 : Inport  Port=11
  Aux4 : Inport  Port=12
  function : TriggerPort  TriggerType=function-call  VariantControl=Variant
  Cast{,1..11} (12 alike) : DataTypeConversion  OutDataTypeStr=uint16
  Mux : Mux  Inputs=12
  Pack_Uart_Message : uartLib/Pack_Uart_Message  SFunctionModules=''
      settings: SourceProductName=GCU Library
  SendUART : uartLib/SendUART  SFunctionModules=''
      settings: SourceProductName=GCU Library
  debugValues : Outport
  wires:
  Mux/1 -> Pack_Uart_Message/1, debugValues/1
  adc_data_vector/1 -> Cast/1
  Cast/1 -> Mux/1
  rpm_Limiter/1 -> Cast1/1
  clutchCurrVal/1 -> Cast2/1
  stateFb/1 -> Cast3/1
  tractionValue/1 -> Cast4/1
  currMode/1 -> Cast5/1
  Aux1/1 -> Cast6/1
  Aux2/1 -> Cast7/1
  Aux3/1 -> Cast8/1
  Aux4/1 -> Cast9/1
  mapValue/1 -> Cast10/1
  Pack_Uart_Message/1 -> SendUART/1
  Cast9/1 -> Mux/12
  Cast8/1 -> Mux/11
  Cast7/1 -> Mux/10
  Cast6/1 -> Mux/9
  Cast10/1 -> Mux/8
  Cast5/1 -> Mux/7
  oil_sensor/1 -> Cast11/1
  Cast4/1 -> Mux/6
  Cast3/1 -> Mux/5
  Cast2/1 -> Mux/4
  Cast1/1 -> Mux/3
  Cast11/1 -> Mux/2

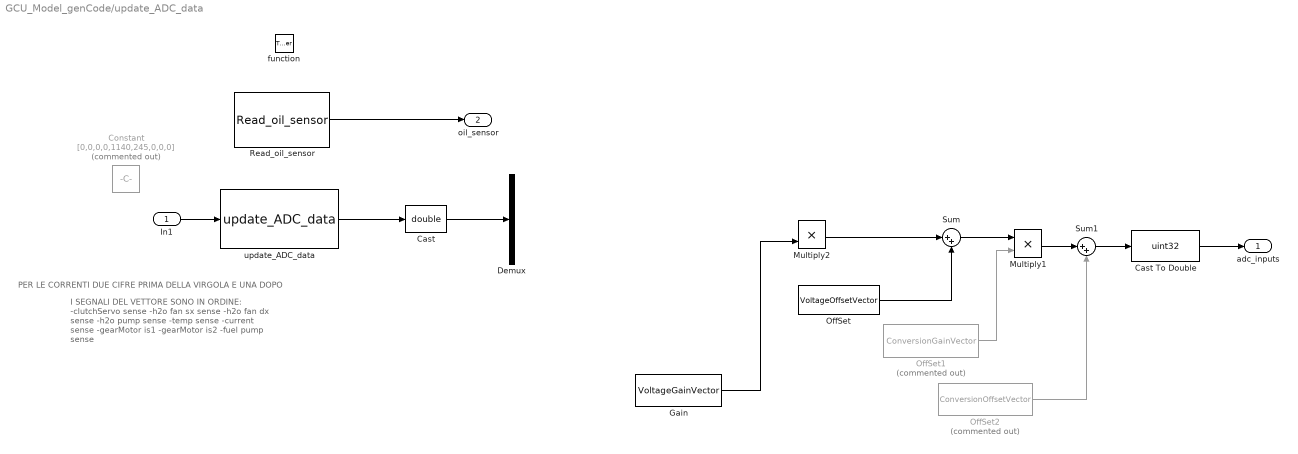
== system GCU_Model_genCode/update_ADC_data ==
  note: I SEGNALI DEL VETTORE SONO IN ORDINE:
      | -clutchServo sense
      | -h2o fan sx sense
      | -h2o fan dx sense
      | -h2o pump sense
      | -temp sense
      | -current sense
      | -gearMotor is1
      | -gearMotor is2
      | -fuel pump sense
  note: PER LE CORRENTI DUE CIFRE PRIMA DELLA VIRGOLA E UNA DOPO
  In1 : Inport
  function : TriggerPort  TriggerType=function-call  VariantControl=Variant
  Cast : DataTypeConversion  OutDataTypeStr=double
  Cast To Double : DataTypeConversion  OutDataTypeStr=uint32
  Constant : Constant  Commented=on  Value=[0,0,0,0,1140,245,0,0,0]  OutDataTypeStr=uint32
  Demux : Demux  Outputs=9
  Gain : Constant  Value=VoltageGainVector  OutDataTypeStr=double
  Multiply1 : Product  OutDataTypeStr=double
  Multiply2 : Product
  OffSet : Constant  Value=VoltageOffsetVector  OutDataTypeStr=double
  OffSet1 : Constant  Commented=on  Value=ConversionGainVector  OutDataTypeStr=double
  OffSet2 : Constant  Commented=on  Value=ConversionOffsetVector  OutDataTypeStr=double
  Read_oil_sensor : S-Function  FunctionName=Read_oil_sensor  SFunctionDeploymentMode=off  EnableBusSupport=off
  Sum : Sum  Inputs=|++
  Sum1 : Sum  Inputs=|++
  update_ADC_data : S-Function  FunctionName=update_ADC_data  SFunctionDeploymentMode=off  EnableBusSupport=off
  adc_inputs : Outport
  oil_sensor : Outport  Port=2
  wires:
  Gain/1 -> Multiply2/2
  update_ADC_data/1 -> Cast/1
  Read_oil_sensor/1 -> oil_sensor/1
  Multiply2/1 -> Sum/1
  OffSet/1 -> Sum/2
  Cast To Double/1 -> adc_inputs/1
  Sum/1 -> Multiply1/1
  OffSet1/1 -> Multiply1/2
  Multiply1/1 -> Sum1/1
  Sum1/1 -> Cast To Double/1
  OffSet2/1 -> Sum1/2
  In1/1 -> update_ADC_data/1
  Cast/1 -> Demux/1

== system GCU_Model_genCode/CAN_Send/Subsystem ==
  id : Inport
  tractionFb : Inport  Port=2
  rpmLimiter : Inport  Port=3
  autogearshiftFb : Inport  Port=4
  stateFb : Inport  Port=5
  function : TriggerPort  TriggerType=function-call  VariantControl=Variant
  sendMessage2 : canLib/sendMessage
      settings: SourceProductName=GCU Library
  wires:
  stateFb/1 -> sendMessage2/5
  id/1 -> sendMessage2/1
  tractionFb/1 -> sendMessage2/2
  rpmLimiter/1 -> sendMessage2/3
  autogearshiftFb/1 -> sendMessage2/4

== system GCU_Model_genCode/CAN_Send/Subsystem1 ==
  id : Inport
  Temp : Inport  Port=2
  gcuCurrent : Inport  Port=3
  h20Pump : Inport  Port=4
  fuelPump : Inport  Port=5
  function : TriggerPort  TriggerType=function-call  VariantControl=Variant
  sendMessage3 : canLib/sendMessage
      settings: SourceProductName=GCU Library
  wires:
  id/1 -> sendMessage3/1
  fuelPump/1 -> sendMessage3/5
  h20Pump/1 -> sendMessage3/4
  Temp/1 -> sendMessage3/2
  gcuCurrent/1 -> sendMessage3/3

== system GCU_Model_genCode/CAN_Send/Subsystem2 ==
  id : Inport
  gearMotorCurrent : Inport  Port=2
  clutchCurrent : Inport  Port=3
  fanSx : Inport  Port=4
  fanDx : Inport  Port=5
  function : TriggerPort  TriggerType=function-call  VariantControl=Variant
  sendMessage4 : canLib/sendMessage
      settings: SourceProductName=GCU Library
  wires:
  id/1 -> sendMessage4/1
  fanSx/1 -> sendMessage4/4
  clutchCurrent/1 -> sendMessage4/3
  gearMotorCurrent/1 -> sendMessage4/2
  fanDx/1 -> sendMessage4/5

== system GCU_Model_genCode/CAN_Send/Subsystem3 ==
  id : Inport
  clutch : Inport  Port=2
  mode : Inport  Port=3
  map : Inport  Port=4
  antiStall : Inport  Port=5
  function : TriggerPort  TriggerType=function-call  VariantControl=Variant
  sendMessage1 : canLib/sendMessage
      settings: SourceProductName=GCU Library
  wires:
  id/1 -> sendMessage1/1
  clutch/1 -> sendMessage1/2
  antiStall/1 -> sendMessage1/5
  map/1 -> sendMessage1/4
  mode/1 -> sendMessage1/3

== system GCU_Model_genCode/CAN_Send/sendMessage ==
  id : Inport
  traction1 : Inport  Port=2
  traction2 : Inport  Port=3
  rpm : Inport  Port=4
  oil : Inport  Port=5
  function : TriggerPort  TriggerType=function-call  VariantControl=Variant
  sendMessage : canLib/sendMessage
      settings: SourceProductName=GCU Library
  wires:
  traction1/1 -> sendMessage/2
  id/1 -> sendMessage/1
  traction2/1 -> sendMessage/3
  oil/1 -> sendMessage/5
  rpm/1 -> sendMessage/4

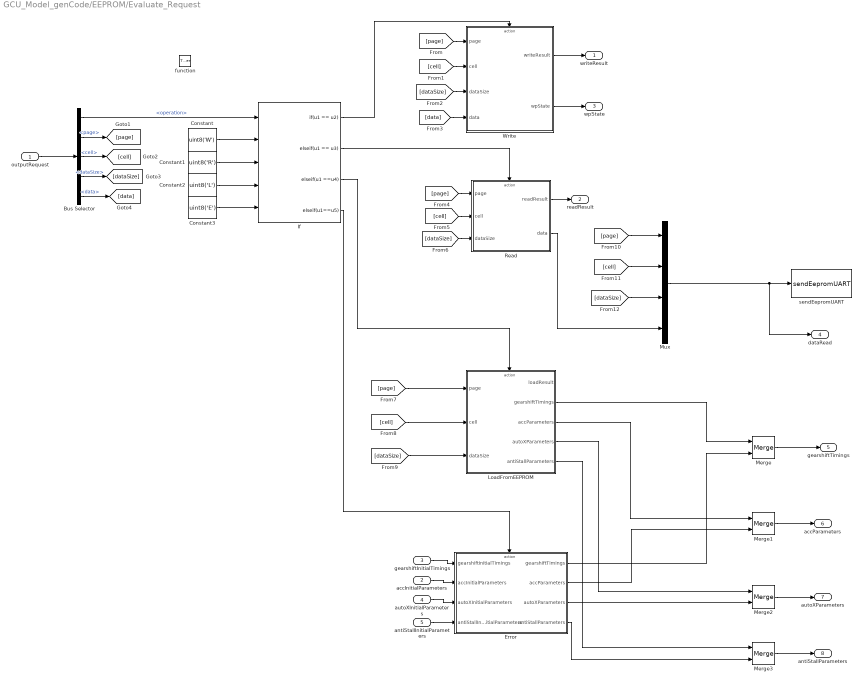
== system GCU_Model_genCode/EEPROM/Evaluate_Request ==
  outputRequest : Inport
  accInitialParameters : Inport  Port=2
  gearshiftInitialTimings : Inport  Port=3
  autoXInitialParameters : Inport  Port=4
  antiStallInitialParameters : Inport  Port=5
  function : TriggerPort  TriggerType=function-call  VariantControl=Variant
  Bus Selector : BusSelector  OutputSignals=operation,page,cell,dataSize,data
  Constant : Constant  Value=uint8('W')  OutDataTypeStr=uint8
  Constant1 : Constant  Value=uint8('R')  OutDataTypeStr=uint8
  Constant2 : Constant  Value=uint8('L')  OutDataTypeStr=uint8
  Constant3 : Constant  Value=uint8('E')  OutDataTypeStr=uint8
  Error : Subsystem  TreatAsAtomicUnit=on
  If : If  NumInputs=5  IfExpression=u1 == u2  ElseIfExpressions=u1 == u3, u1 ==u4, u1==u5  ShowElse=off
  LoadFromEEPROM : Subsystem  TreatAsAtomicUnit=on
  Merge{,1..3} (4 alike) : Merge
  Mux : Mux
  Read : Subsystem  TreatAsAtomicUnit=on
  Write : Subsystem  TreatAsAtomicUnit=on
  sendEepromUART : S-Function  FunctionName=sendEepromUART  SFunctionDeploymentMode=off  EnableBusSupport=off
  writeResult : Outport
  readResult : Outport  Port=2
  wpState : Outport  Port=3
  dataRead : Outport  Port=4  OutDataTypeStr=uint8
  gearshiftTimings : Outport  Port=5
  accParameters : Outport  Port=6
  autoXParameters : Outport  Port=7
  antiStallParameters : Outport  Port=8
  wires:
  outputRequest/1 -> Bus Selector/1
  Constant/1 -> If/2
  Constant1/1 -> If/3
  Write/1(writeResult) -> writeResult/1
  Read/1(readResult) -> readResult/1
  Read/2(data) -> Mux/4
  If/2 -> Read/Action
  If/1 -> Write/Action
  Bus Selector/1 -> If/1  "<operation>"
  Write/2(wpState) -> wpState/1
  Mux/1 -> dataRead/1, sendEepromUART/1
  Constant2/1 -> If/4
  If/3 -> LoadFromEEPROM/Action
  Constant3/1 -> If/5
  If/4 -> Error/Action
  gearshiftInitialTimings/1 -> Error/1(gearshiftInitialTimings)
  Merge/1 -> gearshiftTimings/1
  accInitialParameters/1 -> Error/2(accInitialParameters)
  Merge1/1 -> accParameters/1
  Bus Selector/2 -> [page]  "<page>"
  Bus Selector/3 -> [cell]  "<cell>"
  Bus Selector/4 -> [dataSize]  "<dataSize>"
  Bus Selector/5 -> [data]  "<data>"
  [page] -> Write/1(page)
  [cell] -> Write/2(cell)
  [dataSize] -> Write/3(dataSize)
  [data] -> Write/4(data)
  [page] -> Read/1(page)
  [cell] -> Read/2(cell)
  [dataSize] -> Read/3(dataSize)
  [page] -> LoadFromEEPROM/1(page)
  [cell] -> LoadFromEEPROM/2(cell)
  [dataSize] -> LoadFromEEPROM/3(dataSize)
  [page] -> Mux/1
  [cell] -> Mux/2
  [dataSize] -> Mux/3
  LoadFromEEPROM/2(gearshiftTimings) -> Merge/1
  Error/1(gearshiftTimings) -> Merge/2
  LoadFromEEPROM/3(accParameters) -> Merge1/1
  Error/2(accParameters) -> Merge1/2
  Merge2/1 -> autoXParameters/1
  LoadFromEEPROM/4(autoXParameters) -> Merge2/1
  Error/3(autoXParameters) -> Merge2/2
  autoXInitialParameters/1 -> Error/3(autoXInitialParameters)
  antiStallInitialParameters/1 -> Error/4(antiStallInitialParameters)
  Merge3/1 -> antiStallParameters/1
  LoadFromEEPROM/5(antiStallParameters) -> Merge3/1
  Error/4(antiStallParameters) -> Merge3/2

== system GCU_Model_genCode/GCU_CAN_Read/AAC_ExternalValues ==
  Value : Inport
  Index : Inport  Port=2
  function : TriggerPort  TriggerType=function-call  VariantControl=Variant
  Assignment : Assignment  IndexMode=Zero-based  DiagnosticForDimensions=Warning  IndexOptions=Index vector (port)  Indices=1  OutputSizes=1
  Unit Delay : UnitDelay  InitialCondition=[0,0,0]  SampleTime=-1
  Values : Outport
  wires:
  Assignment/1 -> Unit Delay/1, Values/1
  Unit Delay/1 -> Assignment/1
  Value/1 -> Assignment/2
  Index/1 -> Assignment/3

== system GCU_Model_genCode/GCU_CAN_Read/MessageEvaluation1/setMap ==
  map : Inport  OutDataTypeStr=uint8
  f : TriggerPort  TriggerType=function-call  VariantControl=(inherit)
      settings: CopyFcn=Stateflow.SLINSF.SimulinkMan.removeBlockPreDeleteFcn  PreDeleteFcn=Stateflow.SLINSF.SimulinkMan.unsafePredeleteFcn
  Constant : Constant  OutDataTypeStr=uint8
  Constant1 : Constant  Value=0  OutDataTypeStr=uint8
  If : If  IfExpression=u1 == 1
  If Action Subsystem : Subsystem  TreatAsAtomicUnit=on
  If Action Subsystem1 : Subsystem  TreatAsAtomicUnit=on
  Merge : Merge
  SetMap : S-Function  FunctionName=Efi_setMap  SFunctionDeploymentMode=off  EnableBusSupport=off
  wires:
  Merge/1 -> SetMap/1
  map/1 -> If/1
  If/1 -> If Action Subsystem/Action
  If/2 -> If Action Subsystem1/Action
  Constant/1 -> If Action Subsystem/1(In1)
  If Action Subsystem/1(Out1) -> Merge/1
  Constant1/1 -> If Action Subsystem1/1(In1)
  If Action Subsystem1/1(Out1) -> Merge/2

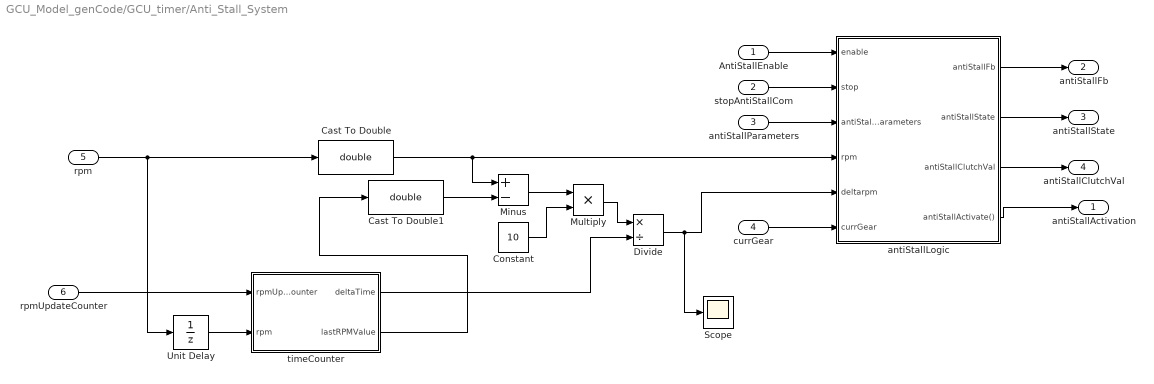
== system GCU_Model_genCode/GCU_timer/Anti_Stall_System ==
  AntiStallEnable : Inport
  stopAntiStallCom : Inport  Port=2
  antiStallParameters : Inport  Port=3
  currGear : Inport  Port=4
  rpm : Inport  Port=5
  rpmUpdateCounter : Inport  Port=6
  Cast To Double : DataTypeConversion  OutDataTypeStr=double
  Cast To Double1 : DataTypeConversion  OutDataTypeStr=double
  Constant : Constant  Value=10
  Divide : Product  Inputs=*/
  Minus : Sum  Inputs=+-
  Multiply : Product
  Scope : Scope
  Unit Delay : UnitDelay  SampleTime=-1
  antiStallLogic : Stateflow chart  TreatAsAtomicUnit=on
  timeCounter : Stateflow chart  TreatAsAtomicUnit=on  SystemSampleTime=0.001
  antiStallActivation : Outport
  antiStallFb : Outport  Port=2
  antiStallState : Outport  Port=3
  antiStallClutchVal : Outport  Port=4
  wires:
  rpm/1 -> Cast To Double/1, Unit Delay/1
  antiStallParameters/1 -> antiStallLogic/3(antiStall_parameters)
  stopAntiStallCom/1 -> antiStallLogic/2(stop)
  AntiStallEnable/1 -> antiStallLogic/1(enable)
  antiStallLogic/4(antiStallActivate()) -> antiStallActivation/1
  antiStallLogic/1(antiStallFb) -> antiStallFb/1
  currGear/1 -> antiStallLogic/6(currGear)
  Constant/1 -> Multiply/2
  Multiply/1 -> Divide/1
  Divide/1 -> Scope/1, antiStallLogic/5(deltarpm)
  rpmUpdateCounter/1 -> timeCounter/1(rpmUpdateCounter)
  timeCounter/1(deltaTime) -> Divide/2
  antiStallLogic/2(antiStallState) -> antiStallState/1
  antiStallLogic/3(antiStallClutchVal) -> antiStallClutchVal/1
  Unit Delay/1 -> timeCounter/2(rpm)
  timeCounter/2(lastRPMValue) -> Cast To Double1/1
  Minus/1 -> Multiply/1
  Cast To Double/1 -> Minus/1, antiStallLogic/4(rpm)
  Cast To Double1/1 -> Minus/2

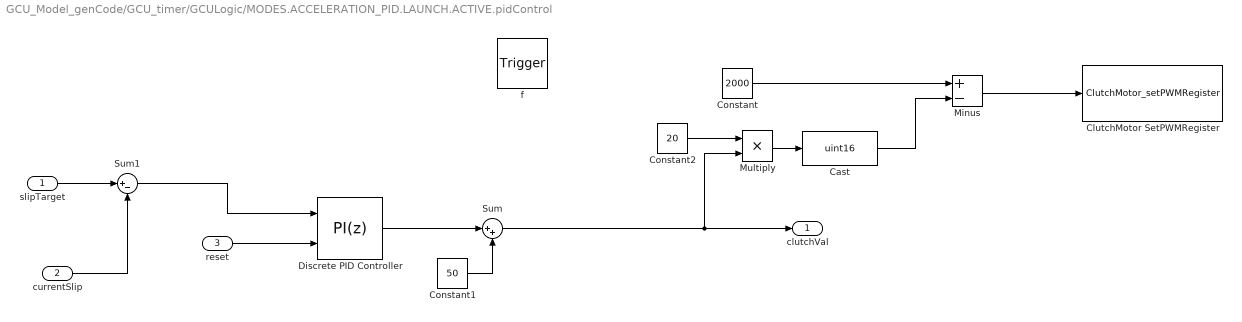
== system GCU_Model_genCode/GCU_timer/GCULogic/MODES.ACCELERATION_PID.LAUNCH.ACTIVE.pidControl ==
  slipTarget : Inport
  currentSlip : Inport  Port=2
  reset : Inport  Port=3
  f : TriggerPort  TriggerType=function-call  VariantControl=(inherit)
      settings: CopyFcn=Stateflow.SLINSF.SimulinkMan.removeBlockPreDeleteFcn  PreDeleteFcn=Stateflow.SLINSF.SimulinkMan.unsafePredeleteFcn
  Cast : DataTypeConversion  OutDataTypeStr=uint16
  ClutchMotor SetPWMRegister : S-Function  FunctionName=ClutchMotor_setPWMRegister  SFunctionDeploymentMode=off  EnableBusSupport=off
  Constant : Constant  Value=2000  OutDataTypeStr=uint16
  Constant1 : Constant  Value=50
  Constant2 : Constant  Value=20  OutDataTypeStr=double
  Discrete PID Controller : simulink/Continuous/PID Controller  Controller=PI  TimeDomain=Discrete-time  SampleTime=-1  IntegratorMethod=Forward Euler  FilterMethod=Forward Euler  Form=Parallel  UseFilter=on  ControllerParametersSource=internal  P=-0.52535095568031  I=-9.79580592329006  D=0.00664206143376672  N=13.2886258278716  InitialConditionSource=internal  InitialConditionForIntegrator=0  InitialConditionForFilter=0  ExternalReset=rising  LimitOutput=on  UpperSaturationLimit=0  LowerSaturationLimit=-50  LinearizeAsGain=off  AntiWindupMode=back-calculation  Kb=1  TrackingMode=off  Kt=1  PParamMin=[]  PParamMax=[]  IParamMin=[]  IParamMax=[]  DParamMin=[]  DParamMax=[]  NParamMin=[]  NParamMax=[]  KbParamMin=[]  KbParamMax=[]  KtParamMin=[]  KtParamMax=[]  POutMin=[]  POutMax=[]  IOutMin=[]  IOutMax=[]  DOutMin=[]  DOutMax=[]  NOutMin=[]  NOutMax=[]  KbOutMin=[]  KbOutMax=[]  KtOutMin=[]  KtOutMax=[]  IntegratorOutMin=[]  IntegratorOutMax=[]  FilterOutMin=[]  FilterOutMax=[]  SumOutMin=[]  SumOutMax=[]  SumI1OutMin=[]  SumI1OutMax=[]  SumI2OutMin=[]  SumI2OutMax=[]  SumI3OutMin=[]  SumI3OutMax=[]  SumDOutMin=[]  SumDOutMax=[]  SaturationOutMin=[]  SaturationOutMax=[]  IntegratorContinuousStateAttributes=''  IntegratorStateMustResolveToSignalObject=off  IntegratorRTWStateStorageClass=Auto  FilterContinuousStateAttributes=''  FilterStateMustResolveToSignalObject=off  FilterRTWStateStorageClass=Auto  DifferentiatorICPrevScaledInput=0  DifferentiatorOutMin=[]  DifferentiatorOutMax=[]  FilterDiffOutCoefMin=[]  FilterDiffOutCoefMax=[]  SumDenOutMin=[]  SumDenOutMax=[]  SumNumOutMin=[]  SumNumOutMax=[]  ReciprocalOutMin=[]  ReciprocalOutMax=[]  DivideOutMin=[]  DivideOutMax=[]  TunerSelectOption=Transfer Function Based (PID Tuner App)
  Minus : Sum  Inputs=+-
  Multiply : Product
  Sum : Sum  Inputs=|++
  Sum1 : Sum  Inputs=|+-
  clutchVal : Outport
  wires:
  currentSlip/1 -> Sum1/2
  Constant/1 -> Minus/1
  Minus/1 -> ClutchMotor SetPWMRegister/1
  Discrete PID Controller/1 -> Sum/1
  Constant1/1 -> Sum/2
  Sum/1 -> Multiply/2, clutchVal/1
  Constant2/1 -> Multiply/1
  Multiply/1 -> Cast/1
  Cast/1 -> Minus/2
  reset/1 -> Discrete PID Controller/2
  slipTarget/1 -> Sum1/1
  Sum1/1 -> Discrete PID Controller/1

== system GCU_Model_genCode/GCU_timer/GCULogic/SCAN_ADC.ScanADC ==
  f : TriggerPort  TriggerType=function-call  VariantControl=(inherit)
      settings: CopyFcn=Stateflow.SLINSF.SimulinkMan.removeBlockPreDeleteFcn  PreDeleteFcn=Stateflow.SLINSF.SimulinkMan.unsafePredeleteFcn
  ScanADC : S-Function  FunctionName=ScanADC  SFunctionDeploymentMode=off  EnableBusSupport=off

== system GCU_Model_genCode/GCU_timer/If Action Subsystem ==
  In1 : Inport
  Action Port : ActionPort  ActionType=then
  Out1 : Outport
  wires:
  In1/1 -> Out1/1

== system GCU_Model_genCode/GCU_timer/If Action Subsystem1 ==
  In1 : Inport
  Action Port : ActionPort  ActionType=else
  Out1 : Outport
  wires:
  In1/1 -> Out1/1

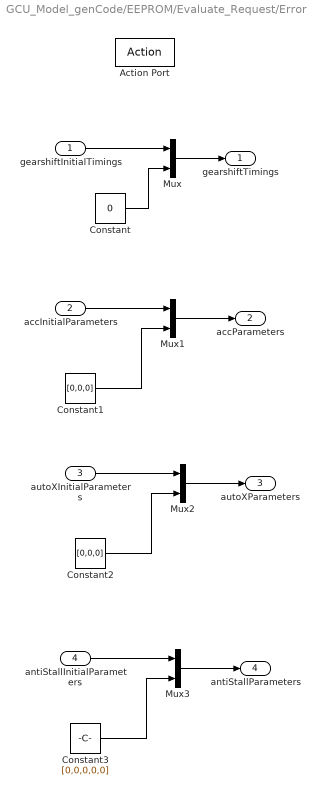
== system GCU_Model_genCode/EEPROM/Evaluate_Request/Error ==
  gearshiftInitialTimings : Inport
  accInitialParameters : Inport  Port=2
  autoXInitialParameters : Inport  Port=3
  antiStallInitialParameters : Inport  Port=4
  Action Port : ActionPort  ActionType=elseif
  Constant : Constant  Value=0  OutDataTypeStr=int32
  Constant1 : Constant  Value=[0,0,0]  OutDataTypeStr=int32
  Constant2 : Constant  Value=[0,0,0]  OutDataTypeStr=int32
  Constant3 : Constant  Value=[0,0,0,0,0]  OutDataTypeStr=int32
  Mux{,1..3} (4 alike) : Mux  Inputs=2
  gearshiftTimings : Outport
  accParameters : Outport  Port=2
  autoXParameters : Outport  Port=3
  antiStallParameters : Outport  Port=4
  wires:
  gearshiftInitialTimings/1 -> Mux/1
  Constant/1 -> Mux/2
  Mux/1 -> gearshiftTimings/1
  Mux1/1 -> accParameters/1
  accInitialParameters/1 -> Mux1/1
  Constant1/1 -> Mux1/2
  Mux2/1 -> autoXParameters/1
  Constant2/1 -> Mux2/2
  autoXInitialParameters/1 -> Mux2/1
  antiStallInitialParameters/1 -> Mux3/1
  Constant3/1 -> Mux3/2
  Mux3/1 -> antiStallParameters/1

== system GCU_Model_genCode/EEPROM/Evaluate_Request/LoadFromEEPROM ==
  page : Inport
  cell : Inport  Port=2
  dataSize : Inport  Port=3
  Action Port : ActionPort  ActionType=elseif
  Cast{1..4} (4 alike) : DataTypeConversion  OutDataTypeStr=int32
  Eeprom_read : S-Function  FunctionName=Eeprom_read  SFunctionDeploymentMode=off  EnableBusSupport=off
  updateValues : Stateflow chart  TreatAsAtomicUnit=on
  loadResult : Outport
  gearshiftTimings : Outport  Port=2
  accParameters : Outport  Port=3
  autoXParameters : Outport  Port=4
  antiStallParameters : Outport  Port=5
  wires:
  Eeprom_read/1 -> updateValues/1(loadResult), loadResult/1
  page/1 -> updateValues/2(page), Eeprom_read/1
  cell/1 -> Eeprom_read/2, updateValues/3(cell)
  dataSize/1 -> updateValues/4(dataSize), Eeprom_read/3
  Eeprom_read/2 -> updateValues/5(data_8bit)
  updateValues/1(gearshiftTimings) -> Cast2/1
  updateValues/2(accParameters) -> Cast3/1
  Cast3/1 -> accParameters/1
  Cast2/1 -> gearshiftTimings/1
  Cast1/1 -> autoXParameters/1
  updateValues/3(autoXParameters) -> Cast1/1
  Cast4/1 -> antiStallParameters/1
  updateValues/4(antiStallParameters) -> Cast4/1
